simulink model "LPV_simulation_2013a"  (R2013a)
settings: Solver=ode5  StartTime=0.0  StopTime=10  FixedStep=1e-3  MaxStep=1e-3  RelTol=1e-3
values from neighbouring files (symbols this model uses):
  Ah = Kopt.Ah    [main.m]
  Bh = Kopt.Bh    [main.m]
  Ch = Kopt.Ch    [main.m]
  Dh = Kopt.Dh    [main.m]
  XY_PD = design_paras.XY_PD    [LPV.m]    (also in main.m = 2)
undefined symbols (not defined in the file or in its folder): Gam_opt, Khinf, sigbuilder_block, Xopt, Yopt
settings Model: Creator=Boran  LastModifiedBy=boran
settings DebuggingCC: UnderspecifiedInitializationDetection=Simplified  MergeDetectMultiDrivingBlocksExec=error  FrameProcessingCompatibilityMsg=error
settings GRTTargetCC: CodeReplacementLibrary=C89/C90 (ANSI)

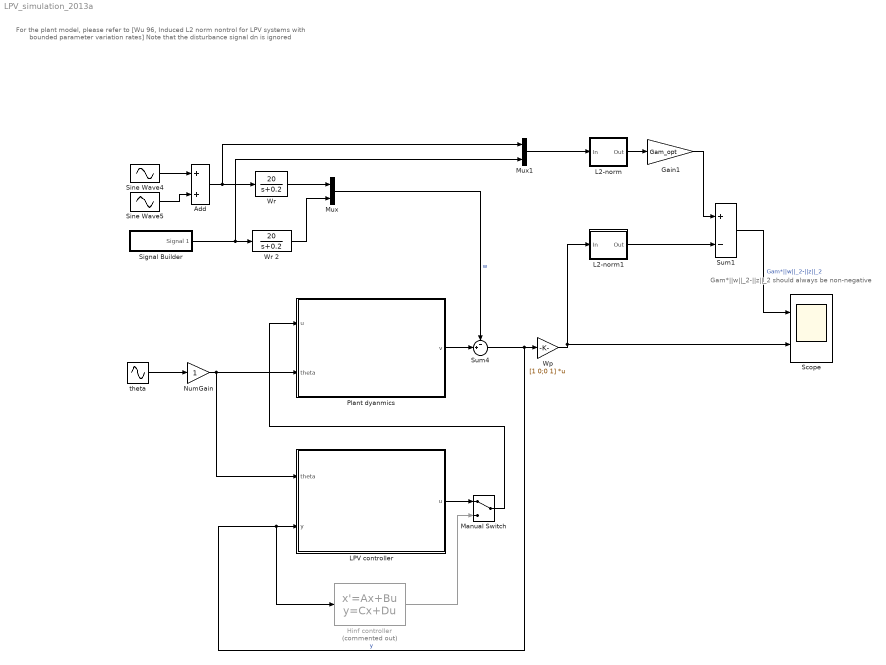
== system LPV_simulation_2013a ==
  note: Gam*||w||_2-||z||_2 should always be non-negative
  note: For the plant model, please refer to [Wu 96, Induced L2 norm nontrol for LPV systems with bounded parameter variation rates]
      | Note that the disturbance signal dn is ignored
  " Wr 2" : TransferFcn  Numerator=[20]  Denominator=[1 0.2]
  Add : Sum
  Gain1 : Gain  Gain=Gam_opt
  Hinf controller : StateSpace  Commented=on  A=Khinf.a  B=Khinf.b  C=Khinf.c  D=Khinf.d  X0=0
  L2-norm : Subsystem
  L2-norm1 : Subsystem
  LPV controller : Subsystem
  Manual Switch : ManualSwitch
  Mux : Mux  Inputs=2
  Mux1 : Mux  Inputs=2
  NumGain : Gain
  Plant dyanmics : Subsystem
  Scope : Scope  NumInputPorts=2
      settings: TimeRange=auto  MaxDataPoints=5000  SaveToWorkspace=off  SaveName=ScopeData  YMin=-0.05016~-0.75424  YMax=0.45141~0.79377  SampleTime=-1
  Signal Builder : Subsystem  Tag=STV Subsys  LoadFcn=sigbuilder_block('load',[437.25 117.75 550.5 394.5 ]);  StartFcn=sigbuilder_block('start');  StopFcn=sigbuilder_block('stop');  ClipboardFcn=sigbuilder_block('clipboard');  mask(Sigbuilder block){}
      mask help: Simulink:masks:SigbuilderBlock_MD
      mask init:
      | if ~strcmp(get_param(bdroot(gcbh),'SimulationStatus'),'stopped') tuvar = sigbuilder_block('maskInit'); end
      settings: CopyFcn=sigbuilder_block('copy');  DeleteFcn=sigbuilder_block('delete');  ModelCloseFcn=sigbuilder_block('modelClose');  PreSaveFcn=sigbuilder_block('preSave');  PauseFcn=sigbuilder_block('pause');  ContinueFcn=sigbuilder_block('continue');  NameChangeFcn=sigbuilder_block('namechange');  OpenFcn=sigbuilder_block('open',[437.25 117.75 550.5 394.5 ]);  CloseFcn=sigbuilder_block('close');
      mask Display: plot(0, 0, 100, 100,[2, 2, 32, 32, 2], [68, 8, 8, 68, 68],[32, 2], [38, 38], [32, 19, 2],[53, 60, 44], [32, 17, 17, 2],[16, 16, 31, 31]);txt = getActiveGroup(gcbh);text(2, 100, txt,'verticalAlignment', 'top');
  Sine Wave4 : Sin  Amplitude=1/2/sqrt(2)  Frequency=2*pi*0.2  SampleTime=0  VectorParams1D=off
  Sine Wave5 : Sin  Amplitude=1/2  Frequency=2*pi*0.5  SampleTime=0
  Sum1 : Sum  Inputs=+-
  Sum4 : Sum  Inputs=-+|
  Wp : Gain  Gain=[1 0;0 1]  Multiplication=Matrix(K*u)
  Wr : TransferFcn  Numerator=[20]  Denominator=[1 0.2]
  theta : Sin  Amplitude=pi  Frequency=5/pi  SampleTime=0
  wires:
  theta/1 -> NumGain/1
  Plant dyanmics/1(v) -> Sum4/2
  Signal Builder/1(Signal 1) -> Mux1/2, " Wr 2"/1
  Mux/1 -> Sum4/1  "w"
  Wr/1 -> Mux/1
  " Wr 2"/1 -> Mux/2
  Sine Wave4/1 -> Add/1
  Sine Wave5/1 -> Add/2
  Add/1 -> Mux1/1, Wr/1
  Sum4/1 -> Hinf controller/1, LPV controller/2(y), Wp/1  "y"
  Mux1/1 -> L2-norm/1(In)
  Wp/1 -> Scope/2, L2-norm1/1(In)
  L2-norm/1(Out) -> Gain1/1
  L2-norm1/1(Out) -> Sum1/2
  Gain1/1 -> Sum1/1
  Sum1/1 -> Scope/1  "Gam*||w||_2-||z||_2"
  Manual Switch/1 -> Plant dyanmics/1(u)
  NumGain/1 -> LPV controller/1(theta), Plant dyanmics/2(theta)
  Hinf controller/1 -> Manual Switch/2
  LPV controller/1(u) -> Manual Switch/1

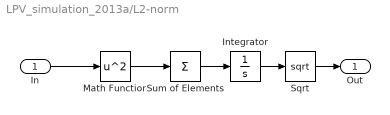
== system LPV_simulation_2013a/L2-norm ==
  In : Inport
  Integrator : Integrator
  Math Function : Math  Operator=square  SaturateOnIntegerOverflow=on
  Sqrt : Sqrt  SaturateOnIntegerOverflow=on
  Sum of Elements : Sum  Inputs=+
  Out : Outport
  wires:
  Sqrt/1 -> Out/1
  Math Function/1 -> Sum of Elements/1
  Sum of Elements/1 -> Integrator/1
  Integrator/1 -> Sqrt/1
  In/1 -> Math Function/1

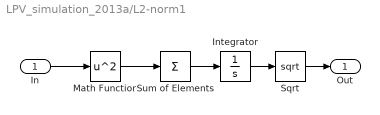
== system LPV_simulation_2013a/L2-norm1 ==
  In : Inport
  Integrator : Integrator
  Math Function : Math  Operator=square  SaturateOnIntegerOverflow=on
  Sqrt : Sqrt  SaturateOnIntegerOverflow=on
  Sum of Elements : Sum  Inputs=+
  Out : Outport
  wires:
  In/1 -> Math Function/1
  Integrator/1 -> Sqrt/1
  Sum of Elements/1 -> Integrator/1
  Math Function/1 -> Sum of Elements/1
  Sqrt/1 -> Out/1

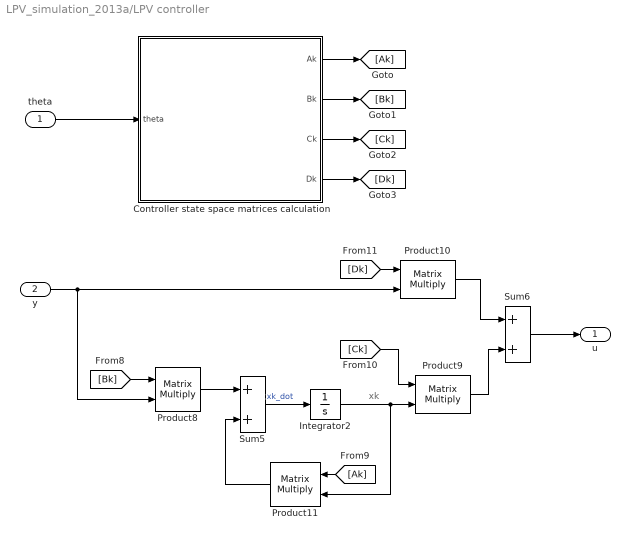
== system LPV_simulation_2013a/LPV controller ==
  note: xk
  theta : Inport
  y : Inport  Port=2
  "Controller state space matrices calculation " : MATLAB Function  TreatAsAtomicUnit=on
      settings: PermitHierarchicalResolution=ParametersOnly  MinAlgLoopOccurrences=on
  Integrator2 : Integrator
  Product{8..11} (4 alike) : Product  Multiplication=Matrix(*)
  Sum5 : Sum
  Sum6 : Sum
  u : Outport
  wires:
  Product11/1 -> Sum5/2
  [Dk] -> Product10/1
  y/1 -> Product10/2, Product8/2
  Product9/1 -> Sum6/2
  [Bk] -> Product8/1
  [Ak] -> Product11/1
  Product8/1 -> Sum5/1
  Sum5/1 -> Integrator2/1  "xk_dot"
  [Ck] -> Product9/1
  Integrator2/1 -> Product9/2, Product11/2
  Sum6/1 -> u/1
  Product10/1 -> Sum6/1
  theta/1 -> "Controller state space matrices calculation "/1(theta)
  "Controller state space matrices calculation "/3(Ck) -> [Ck]
  "Controller state space matrices calculation "/4(Dk) -> [Dk]
  "Controller state space matrices calculation "/1(Ak) -> [Ak]
  "Controller state space matrices calculation "/2(Bk) -> [Bk]

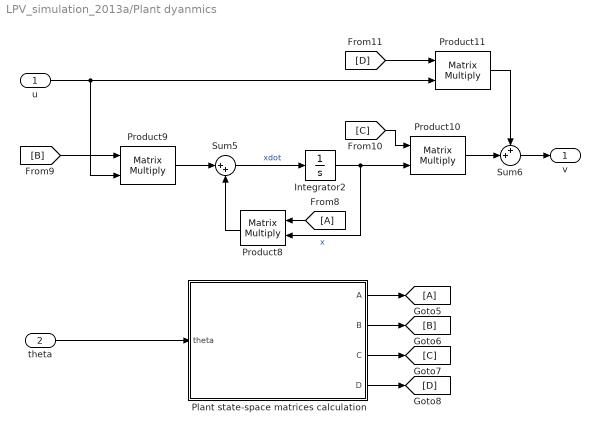
== system LPV_simulation_2013a/Plant dyanmics ==
  u : Inport
  theta : Inport  Port=2
  Integrator2 : Integrator
  Plant state-space matrices calculation : MATLAB Function  TreatAsAtomicUnit=on
      settings: PermitHierarchicalResolution=ParametersOnly  MinAlgLoopOccurrences=on
  Product{8..11} (4 alike) : Product  Multiplication=Matrix(*)
  Sum5 : Sum  Inputs=|++
  Sum6 : Sum  Inputs=++|
  v : Outport
  wires:
  Plant state-space matrices calculation/1(A) -> [A]
  Plant state-space matrices calculation/2(B) -> [B]
  Plant state-space matrices calculation/3(C) -> [C]
  Plant state-space matrices calculation/4(D) -> [D]
  u/1 -> Product11/2, Product9/2
  Integrator2/1 -> Product10/2, Product8/2  "x"
  [D] -> Product11/1
  [C] -> Product10/1
  Product11/1 -> Sum6/1
  Product8/1 -> Sum5/2
  Product9/1 -> Sum5/1
  Sum5/1 -> Integrator2/1  "xdot"
  [A] -> Product8/1
  [B] -> Product9/1
  Product10/1 -> Sum6/2
  Sum6/1 -> v/1
  theta/1 -> Plant state-space matrices calculation/1(theta)

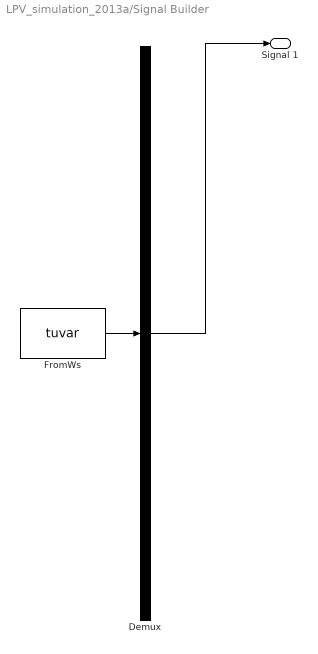
== system LPV_simulation_2013a/Signal Builder ==
  Demux : Demux  Tag=STV Demux  Outputs=1
  FromWs : FromWorkspace  Tag=STV FromWs  VariableName=tuvar  SampleTime=0
      SigBuilderData=|
      | common.afterFinalStr = 'Extrapolate'
      | common.sampleTime = 0
      | dataSet.timeRange = [0 10]
      | dataSet.name = 'Group 1'
      | sbobj.Groups.Name = 'Group 1'
      | sbobj.Groups.Signals.Name = 'Signal 1'
      | sbobj.Groups.Signals.XData = [0 1 2 3.5 5 7.5 10]
      | sbobj.Groups.Signals.YData = [0 0.707106781187 0.71 -0.5 -0.495 0 0]
  Signal 1 : Outport  Tag=STV Outport
  wires:
  Demux/1 -> Signal 1/1
  FromWs/1 -> Demux/1

== matlab function LPV_simulation_2013a/LPV controller/Controller state space matrices calculation  ==
  data: theta input; Xopt parameter; Yopt parameter; Ak output; Bk output; Ck output; Dk output; Ah parameter; Bh parameter; Ch parameter; Dh parameter; XY_PD parameter
function [Ak, Bk, Ck, Dk] = Controller(theta,Xopt, Yopt, Ah, Bh, Ch, Dh, XY_PD)

% The following code should be customized for each example.

% global Khatopt Xopt Yopt  
 A = [0.75 2 cos(theta) sin(theta) 0 0;...
     0 0.5 -sin(theta) cos(theta) 0 0;...
     0 0 -10 0 0 0;...
     0 0 0 -10 0 0;...
     0 0 0 0 -0.2 0;
     0 0 0 0 0 -0.2];
 B2 = [0 0; 0 0;10 0; 0 10;0 0; 0 0];
 C2 = [1 0 0 0 -5 0;0 1 0 0 0 -5];

Ftheta = [1 cos(theta) sin(theta)];
I = eye(size(Xopt,1));
% Note that any M, N satisfying N*M' = I - XY can be selected
if XY_PD == 1  
    X = Xopt(:,:,1) + cos(theta)*Xopt(:,:,2) + sin(theta)*Xopt(:,:,3);
    Y = Yopt(:,:,1);
%     DX = -sin(theta)*Xopt(:,:,2) + cos(theta)*Xopt(:,:,3);
    % X*Ydot +N*Mdot' = 0
%     M = -Y;
%     N = X - I/Y;      
      M = I;
      N = I - X*Y;
elseif XY_PD == 2
    Y = Yopt(:,:,1) + Ftheta(2)*Yopt(:,:,2) + Ftheta(3)*Yopt(:,:,3);
    X = Xopt(:,:,1);
    % Xdot*Y + Ndot*M' = 0
%     N = -X;
%     M = Y - I/X;
    N = I;
    M = I - Y*X;
else % XY_PD == 0
    Y = Yopt(:,:,1);
    X = Xopt(:,:,1);
%     N = -X;
%     M = Y - I/X;
    N = I;
    M = I - Y*X;
end
Akhat = Ah(:,:,1) + Ftheta(2)*Ah(:,:,2) + Ftheta(3)*Ah(:,:,3);
Bkhat = Bh(:,:,1) + Ftheta(2)*Bh(:,:,2) + Ftheta(3)*Bh(:,:,3);
Ckhat = Ch(:,:,1) + Ftheta(2)*Ch(:,:,2) + Ftheta(3)*Ch(:,:,3);
Dkhat = Dh(:,:,1) + Ftheta(2)*Dh(:,:,2) + Ftheta(3)*Dh(:,:,3);

Dk = Dkhat;
Ck = (Ckhat - Dk*C2*Y)/M';
Bk = N\(Bkhat - X*B2*Dk);
Ak = N\(Akhat - Bkhat*C2*Y - X*B2*Ckhat - X*(A-B2*Dk*C2)*Y)/M';
end

== matlab function LPV_simulation_2013a/Plant dyanmics/Plant state-space matrices calculation ==
  data: theta input; A output; B output; C output; D output
function [A,B,C,D] = Plant(theta)
%#codegen
A = [0.75 2 cos(theta) sin(theta);...
     0 0.5 -sin(theta) cos(theta);...
     0 0 -10 0;...
     0 0 0 -10];
B = [0 0; 0 0;10 0; 0 10];
C = [1 0 0 0;0 1 0 0];
D = [0 0;0 0];
end
